simulink model "regler_sat_isep_mdl"  (R2013b)
settings: Solver=ode45  StartTime=0.0  StopTime=0.5  RelTol=1e-3
values from neighbouring files (symbols this model uses):
  K = 0.05    [regler_sat_isep.m]
  Kg = K / (K*K + a*R)    (= 16.6666666667)    [regler_sat_isep.m]
  Kp = 1    [regler_sat_isep.m]
  mmax = 0.00    (= 0)    [regler_sat_isep.m]
  R = 0.5    [regler_sat_isep.m]
  tau = J*R / (K*K + a*R)    (= 0.0416666666667)    [regler_sat_isep.m]
  Ti = tau    (= 0.0416666666667)    [regler_sat_isep.m]
settings Model: Creator=daniw  LastModifiedBy=daniw
settings DataIOCC: LimitDataPoints=off

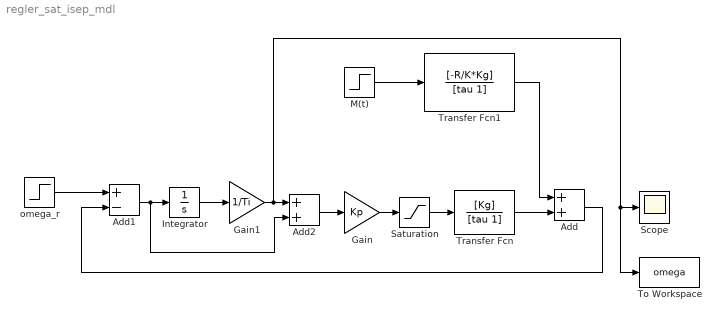
== system regler_sat_isep_mdl ==
  Add : Sum
  Add1 : Sum  Inputs=+-
  Add2 : Sum
  Gain : Gain  Gain=Kp
  Gain1 : Gain  Gain=1/Ti
  Integrator : Integrator
  M(t) : Step  Time=2  After=mmax  SampleTime=0
  Saturation : Saturate  UpperLimit=10  LowerLimit=-10
  Scope : Scope
  To Workspace : ToWorkspace  VariableName=omega  SampleTime=-1  SaveFormat=Structure With Time
  Transfer Fcn : TransferFcn  Numerator=[Kg]  Denominator=[tau 1]
  Transfer Fcn1 : TransferFcn  Numerator=[-R/K*Kg]  Denominator=[tau 1]
  omega_r : Step  Time=0.1  Before=50  After=100  SampleTime=0
  wires:
  M(t)/1 -> Transfer Fcn1/1
  omega_r/1 -> Add1/1
  Add/1 -> Add1/2
  Transfer Fcn/1 -> Add/2
  Transfer Fcn1/1 -> Add/1
  Gain/1 -> Saturation/1
  Add1/1 -> Add2/2, Integrator/1
  Integrator/1 -> Gain1/1
  Add2/1 -> Gain/1
  Gain1/1 -> To Workspace/1, Scope/1, Add2/1
  Saturation/1 -> Transfer Fcn/1
